simulink model "Requriment_2"  (R2021a)
settings: Solver=FixedStepDiscrete  StartTime=0.0  StopTime=17  FixedStep=1  RelTol=1e-3
libraries: simulink x6
settings Model: Creator=Admin  LastModifiedBy=Rahul
settings SolverCC: AlgebraicLoopSolver=TrustRegion
settings OptimizationCC: DefaultParameterBehavior=Inlined  UseDivisionForNetSlopeComputation=on  GainParamInheritBuiltInType=on  UseFloatMulNetSlope=on  InlineInvariantSignals=on  PassReuseOutputArgsAs=Individual arguments  ZeroExternalMemoryAtStartup=off  ZeroInternalMemoryAtStartup=off  NoFixptDivByZeroProtection=on  EfficientFloat2IntCast=on  LifeSpan=1  OptimizeBlockOrder=speed  DifferentSizesBufferReuse=on  EfficientTunableParamExpr=on
settings DebuggingCC: SignalInfNanChecking=error  ParameterTunabilityLossMsg=error  UniqueDataStoreMsg=error  AssertControl=DisableAll  StrictBusMsg=ErrorOnBusTreatedAsVector  SFUndirectedBroadcastEventsDiag=error  SFMachineParentedDataDiag=warning
settings HardwareCC: ProdLongLongMode=on
settings SFSimCC: CompileTimeRecursionLimit=0  EnableRuntimeRecursion=off  MATLABDynamicMemAlloc=off  CustomCodeUndefinedFunction=UseInterfaceOnly
settings RTWCC: SystemTargetFile=ert.tlc  TemplateMakefile=ert_default_tmf  GenerateReport=on  IncludeHyperlinkInReport=on  LaunchReport=on  GenerateTraceInfo=on  GenerateTraceReport=on  GenerateTraceReportSl=on  GenerateTraceReportSf=on  GenerateTraceReportEml=on  GenerateCodeMetricsReport=on
settings CodeAppCC: ForceParamTrailComments=on  IgnoreCustomStorageClasses=off  OperatorAnnotations=on  SimulinkDataObjDesc=on  SFDataObjDesc=on  MATLABFcnDesc=on  CustomSymbolStrGlobalVar=rt$N$M  CustomSymbolStrType=$N$M  CustomSymbolStrFcn=$N$M$F  CustomSymbolStrMacro=$N$M  InsertBlockDesc=on
settings ERTTargetCC: TargetLangStandard=C99 (ISO)  UtilityFuncGeneration=Shared location  GenerateSampleERTMain=on  IncludeMdlTerminateFcn=off  CombineSignalStateStructs=on  SupportAbsoluteTime=off  SupportNonFinite=off  SupportComplex=off  ParenthesesLevel=Maximum  CastingMode=Standards  GenerateSharedConstants=off  InlinedParameterPlacement=NonHierarchical  ERTCustomFileTemplate=example_file_process.tlc  ERTFilePackagingFormat=CompactWithDataFile  EnableSignedLeftShifts=off  EnableSignedRightShifts=off
settings ConfigComp: CovMetricSettings=dcmwe  DVTestSuiteOptimization=Auto  DVDetectDeadLogic=on  DVDetectOutOfBounds=on  DVDataFileName=re2  DVSaveReport=on  DVReportFileName=re2_report  DVRebuildModelRepresentation=Always

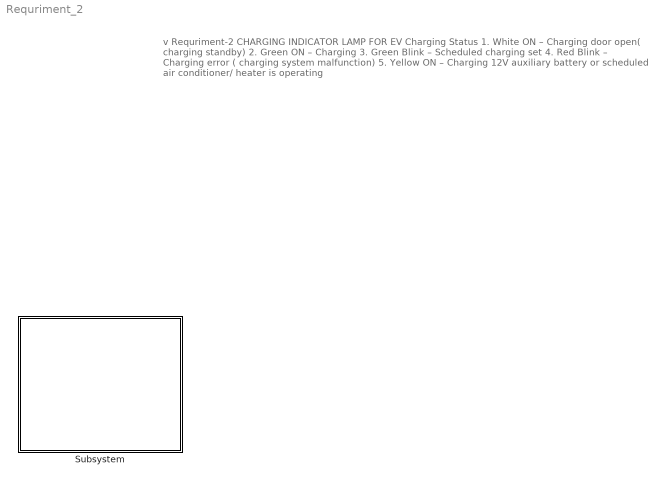
== system Requriment_2 ==
  note: v Requriment-2
      | CHARGING INDICATOR LAMP FOR EV
      | Charging Status
      | 1. White ON – Charging door open( charging standby)
      | 2. Green ON – Charging
      | 3. Green Blink – Scheduled charging set
      | 4. Red Blink – Charging error ( charging system malfunction)
      | 5. Yellow ON – Charging 12V auxiliary battery or scheduled air conditioner/ heater is operating
  Subsystem : Subsystem  TreatAsAtomicUnit=on

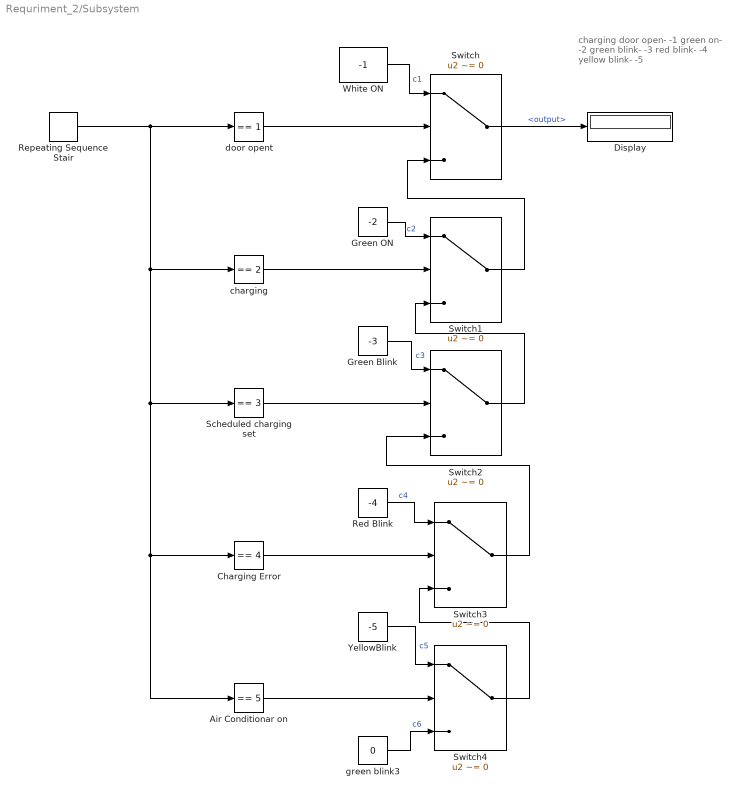
== system Requriment_2/Subsystem ==
  note: charging door open- -1
      | green on- -2
      | green blink-  -3
      | red blink- -4
      | yellow blink- -5
  "Air Conditionar on " : simulink/Logic and Bit Operations/Compare To Constant  relop===  const=5  OutDataTypeStr=boolean
  Charging Error : simulink/Logic and Bit Operations/Compare To Constant  relop===  const=4  OutDataTypeStr=boolean
  Display : Display
  Green Blink : Constant  Value=-3
  Green ON : Constant  Value=-2
  Red Blink : Constant  Value=-4
  Repeating Sequence Stair : simulink/Sources/Repeating Sequence Stair  OutValues=[0 1 3 5 3 2 5 1 4 1 3 5]  tsamp=-1  OutMin=[]  OutMax=[]  OutDataTypeStr=double  OutputDataTypeScalingMode=double  OutDataType=fixdt(0,8)  ConRadixGroup=Best Precision: Vector-wise  OutScaling=2^-12
  "Scheduled charging set " : simulink/Logic and Bit Operations/Compare To Constant  relop===  const=3  OutDataTypeStr=boolean
  Switch{,1..4} (5 alike) : Switch  Criteria=u2 ~= 0
  White ON : Constant  Value=-1
  YellowBlink : Constant  Value=-5
  charging : simulink/Logic and Bit Operations/Compare To Constant  relop===  const=2  OutDataTypeStr=boolean
  door opent : simulink/Logic and Bit Operations/Compare To Constant  relop===  const=1  OutDataTypeStr=boolean
  green blink3 : Constant  Value=0
  wires:
  White ON/1 -> Switch/1  "c1"
  "Scheduled charging set "/1 -> Switch2/2
  Repeating Sequence Stair/1 -> "Air Conditionar on "/1, Charging Error/1, "Scheduled charging set "/1, charging/1, door opent/1
  Switch/1 -> Display/1  "<output>"
  Green Blink/1 -> Switch2/1  "c3"
  Switch3/1 -> Switch2/3
  door opent/1 -> Switch/2
  Switch2/1 -> Switch1/3
  charging/1 -> Switch1/2
  Switch1/1 -> Switch/3
  Green ON/1 -> Switch1/1  "c2"
  Red Blink/1 -> Switch3/1  "c4"
  Switch4/1 -> Switch3/3
  Charging Error/1 -> Switch3/2
  YellowBlink/1 -> Switch4/1  "c5"
  green blink3/1 -> Switch4/3  "c6"
  "Air Conditionar on "/1 -> Switch4/2
